simulink model "CMG_Model"  (R2025a)
settings: Solver=VariableStepAuto  StartTime=0.0  StopTime=320  RelTol=1e-3
values from neighbouring files (symbols this model uses):
  J = Jm + Jdisk    (= 1.0323014)    [Reaction_Wheel_Model_Variables.m]
  Js = 0.0022    [Reaction_Wheel_Model_Variables.m]
  Kta = 1    [Reaction_Wheel_Model_Variables.m]
  omegas = 209.44    [Reaction_Wheel_Model_Variables.m]
libraries: simulink_extras x2
settings Model: Creator=Stefan1  LastModifiedBy=Stefan1

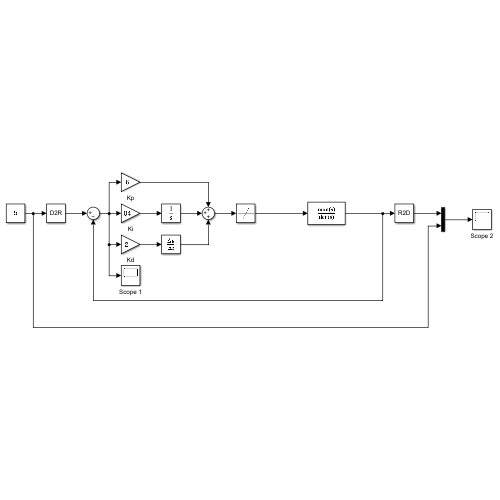
[thumbnail: Simulink's stored preview of the top-level diagram]
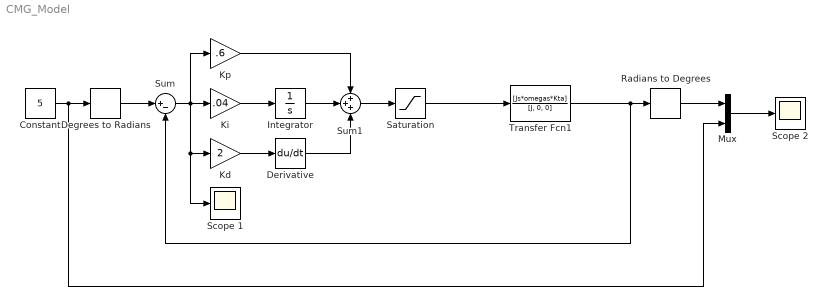
== system CMG_Model ==
  Constant : Constant  Value=5
  Degrees to Radians : simulink_extras/Transformations/Degrees to Radians
  Derivative : Derivative
  Integrator : Integrator
  Kd : Gain  Gain=2
  Ki : Gain  Gain=.04
  Kp : Gain  Gain=.6
  Mux : Mux  Inputs=2
  Radians to Degrees : simulink_extras/Transformations/Radians to Degrees
  Saturation : Saturate  UpperLimit=12  LowerLimit=-12
  Scope 1 : Scope
      settings: ActiveDisplayYMinimum=-0.85098149542235213  ActiveDisplayYMaximum=0.64921398545764364
  Scope 2 : Scope
      settings: ActiveDisplayYMinimum=-9.9503505803806185  ActiveDisplayYMaximum=89.553155223425577
  Sum : Sum  Inputs=|+-
  Sum1 : Sum  Inputs=+++
  Transfer Fcn1 : TransferFcn  Numerator=[Js*omegas*Kta]  Denominator=[J, 0, 0]
  wires:
  Kd/1 -> Derivative/1
  Ki/1 -> Integrator/1
  Integrator/1 -> Sum1/2
  Sum1/1 -> Saturation/1
  Constant/1 -> Mux/2, Degrees to Radians/1
  Degrees to Radians/1 -> Sum/1
  Sum/1 -> Scope 1/1, Kd/1, Kp/1, Ki/1
  Kp/1 -> Sum1/1
  Derivative/1 -> Sum1/3
  Saturation/1 -> Transfer Fcn1/1
  Transfer Fcn1/1 -> Sum/2, Radians to Degrees/1
  Radians to Degrees/1 -> Mux/1
  Mux/1 -> Scope 2/1
